simulink model "Discrete_Adaptive_Saturation"  (R2016b)
settings: Solver=FixedStepAuto  StartTime=0.0  StopTime=60  FixedStep=Ts  RelTol=1e-3
values from neighbouring files (symbols this model uses):
  A = [0 1;0 0]    [Adaptive.m]
  Am = [-2*xim*wm -wm^2;1 0]    [Adaptive.m]
  B = [0;K]    [Adaptive.m]
  Bm = [1;0]    [Adaptive.m]
  C = [1 0]    [Adaptive.m]
  Cm = [0 wm^2]    [Adaptive.m]
  D = 0    [Adaptive.m]
  Dm = 0    [Adaptive.m]
  down = -up    (= -0.0872664625997)    [Adaptive.m]
  gammar = 1    [Adaptive.m]
  gammax = diag([35 10])    [Adaptive.m]
  P_bar = [double(S.p12);double(S.p22)]    [Adaptive.m]
  Ts = 0.01    [Adaptive.m]
  up = 5*pi/180    (= 0.0872664625997)    [Adaptive.m]
undefined symbols (not defined in the file or in its folder): DiscIntNeverNeededParam
libraries: simulink x6
settings Model: Creator=Ashraf  LastModifiedBy=Ashraf

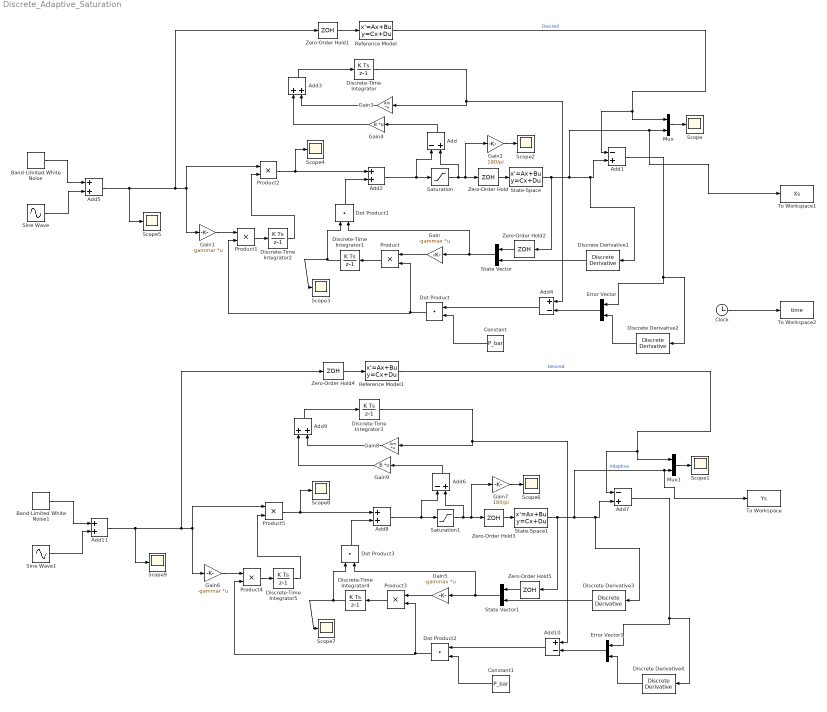
== system Discrete_Adaptive_Saturation ==
  Add{,1,6..7} (4 alike) : Sum  Inputs=-+
  Add10 : Sum  Inputs=+-
  Add{2..3,5,8..9,11} (6 alike) : Sum
  Add4 : Sum  Inputs=+-
  Band-Limited White Noise : simulink/Sources/Band-Limited White Noise  Cov=0.00001  Ts=Ts  seed=[23341]
  Band-Limited White Noise1 : simulink/Sources/Band-Limited White Noise  Cov=0.00001  Ts=Ts  seed=[23341]
  Clock : Clock
  Constant : Constant  Value=P_bar
  Constant1 : Constant  Value=P_bar
  Discrete Derivative{1..4} (4 alike) : simulink/Discrete/Discrete Derivative  gainval=1.0  ICPrevScaledInput=0.0  OutMin=[]  OutMax=[]  OutDataType=fixdt(1, 16)  OutScaling=2^-10  DoSatur=off
  Discrete-Time Integrator{,1..5} (6 alike) : DiscreteIntegrator  InitialConditionSetting=State (most efficient)  SampleTime=Ts  ICPrevOutput=DiscIntNeverNeededParam  ICPrevScaledInput=DiscIntNeverNeededParam
  Dot Product{,1..3} (4 alike) : DotProduct  InputSameDT=on  OutDataTypeStr=Inherit: Inherit via internal rule
  Error Vector : Concatenate
  Error Vector1 : Concatenate
  Gain : Gain  Gain=-gammax  Multiplication=Matrix(K*u)
  Gain1 : Gain  Gain=-gammar  Multiplication=Matrix(K*u)
  Gain2 : Gain  Gain=180/pi
  Gain3 : Gain  Gain=Am  Multiplication=Matrix(K*u)
  Gain4 : Gain  Gain=B  Multiplication=Matrix(K*u)
  Gain5 : Gain  Gain=-gammax  Multiplication=Matrix(K*u)
  Gain6 : Gain  Gain=-gammar  Multiplication=Matrix(K*u)
  Gain7 : Gain  Gain=180/pi
  Gain8 : Gain  Gain=Am  Multiplication=Matrix(K*u)
  Gain9 : Gain  Gain=B  Multiplication=Matrix(K*u)
  Mux : Mux  Inputs=2
  Mux1 : Mux  Inputs=2
  Product{,1..5} (6 alike) : Product
  Reference Model : StateSpace  A=Am  B=Bm  C=Cm  D=Dm  X0=[0 0]
  Reference Model1 : StateSpace  A=Am  B=Bm  C=Cm  D=Dm  X0=[0 0]
  Saturation : Saturate  UpperLimit=up  LowerLimit=down
  Saturation1 : Saturate  UpperLimit=up  LowerLimit=down
  Scope{,1..9} (10 alike) : Scope
  Sine Wave : Sin  Amplitude=0.2  Phase=pi/2  SampleTime=Ts
  Sine Wave1 : Sin  Amplitude=0.2  SampleTime=Ts
  State Vector : Concatenate
  State Vector1 : Concatenate
  State-Space : StateSpace  A=A  B=B  C=C  D=D  X0=[0 0]
  State-Space1 : StateSpace  A=A  B=B  C=C  D=D  X0=[0 0]
  To Workspace : ToWorkspace  VariableName=Ys  SampleTime=Ts
  To Workspace1 : ToWorkspace  VariableName=Xs  SampleTime=Ts
  To Workspace2 : ToWorkspace  VariableName=time  SampleTime=Ts
  Zero-Order Hold{,1..5} (6 alike) : ZeroOrderHold  SampleTime=Ts
  wires:
  Add5/1 -> Scope5/1, Gain1/1, Product2/1, Zero-Order Hold1/1
  Reference Model/1 -> Add1/1, Mux/1  "Desired"
  Add1/1 -> Discrete Derivative2/1, Error Vector/1
  Discrete Derivative2/1 -> Error Vector/2
  Constant/1 -> Dot Product/2
  Discrete Derivative1/1 -> State Vector/2
  State Vector/1 -> Dot Product1/2, Gain/1
  Dot Product/1 -> Product/2, Product1/2
  Gain/1 -> Product/1
  Product/1 -> Discrete-Time Integrator1/1
  Discrete-Time Integrator1/1 -> Scope3/1, Dot Product1/1
  Gain1/1 -> Product1/1
  Product1/1 -> Discrete-Time Integrator2/1
  Discrete-Time Integrator2/1 -> Product2/2
  Product2/1 -> Scope4/1, Add2/1
  Dot Product1/1 -> Add2/2
  Gain2/1 -> Scope2/1
  Add2/1 -> Add/1, Saturation/1
  Mux/1 -> Scope/1
  Saturation/1 -> Add/2, Zero-Order Hold/1, Gain2/1
  Add/1 -> Gain4/1
  Gain3/1 -> Add3/2
  Gain4/1 -> Add3/1
  Add3/1 -> Discrete-Time Integrator/1
  Error Vector/1 -> Add4/2
  Discrete-Time Integrator/1 -> Add4/1, Gain3/1
  Add4/1 -> Dot Product/1
  Zero-Order Hold/1 -> State-Space/1
  Zero-Order Hold1/1 -> Reference Model/1
  Zero-Order Hold2/1 -> State Vector/1
  Sine Wave/1 -> Add5/2
  Band-Limited White Noise/1 -> Add5/1
  State-Space1/1 -> To Workspace/1, Mux1/2, Discrete Derivative3/1, Add7/2, Zero-Order Hold5/1  "Adaptive"
  Add11/1 -> Scope9/1, Gain6/1, Product5/1, Zero-Order Hold4/1
  Reference Model1/1 -> Add7/1, Mux1/1  "Desired"
  Add7/1 -> Discrete Derivative4/1, Error Vector1/1
  Discrete Derivative4/1 -> Error Vector1/2
  Constant1/1 -> Dot Product2/2
  Discrete Derivative3/1 -> State Vector1/2
  State Vector1/1 -> Dot Product3/2, Gain5/1
  Dot Product2/1 -> Product3/2, Product4/2
  Gain5/1 -> Product3/1
  Product3/1 -> Discrete-Time Integrator4/1
  Discrete-Time Integrator4/1 -> Scope7/1, Dot Product3/1
  Gain6/1 -> Product4/1
  Product4/1 -> Discrete-Time Integrator5/1
  Discrete-Time Integrator5/1 -> Product5/2
  Product5/1 -> Scope8/1, Add8/1
  Dot Product3/1 -> Add8/2
  Gain7/1 -> Scope6/1
  Add8/1 -> Add6/1, Saturation1/1
  Mux1/1 -> Scope1/1
  Saturation1/1 -> Add6/2, Zero-Order Hold3/1, Gain7/1
  Add6/1 -> Gain9/1
  Gain8/1 -> Add9/2
  Gain9/1 -> Add9/1
  Add9/1 -> Discrete-Time Integrator3/1
  Error Vector1/1 -> Add10/2
  Discrete-Time Integrator3/1 -> Add10/1, Gain8/1
  Add10/1 -> Dot Product2/1
  Zero-Order Hold3/1 -> State-Space1/1
  Zero-Order Hold4/1 -> Reference Model1/1
  Zero-Order Hold5/1 -> State Vector1/1
  Sine Wave1/1 -> Add11/2
  Band-Limited White Noise1/1 -> Add11/1
  State-Space/1 -> To Workspace1/1, Mux/2, Discrete Derivative1/1, Add1/2, Zero-Order Hold2/1
  Clock/1 -> To Workspace2/1
